simulink model "Ackermann"  (Simulink 8.7)
settings: Solver=ode45  StartTime=0.0  StopTime=10.0  RelTol=1e-3
settings Model: Creator=scaife  LastModifiedBy=bourbouh  ExtModeAutoUpdateStatusClock=off
settings DataIOCC: SignalLoggingSaveFormat=ModelDataLogs  SignalLoggingName=sigsOut
settings DebuggingCC: SaveWithParameterizedLinksMsg=none  SignalResolutionControl=TryResolveAllWithWarning  MultiTaskDSMMsg=warning  MultiTaskCondExecSysMsg=none  StrictBusMsg=None
settings HardwareCC: TargetUnknown=on
settings SFSimCC: SimParseCustomCode=off
settings GRTTargetCC: GeneratePreprocessorConditionals=Use local settings  CombineOutputUpdateFcns=off  GRTInterface=on

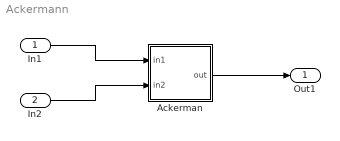
== system Ackermann ==
  In1 : Inport
  In2 : Inport  Port=2
  Ackerman : Stateflow chart  TreatAsAtomicUnit=on
  Out1 : Outport
  wires:
  Ackerman/1(out) -> Out1/1
  In1/1 -> Ackerman/1(in1)
  In2/1 -> Ackerman/2(in2)

== stateflow chart Ackerman ==
  state A/
    entry:
    x[1]=in1;
    y[1]=in2;
    mode[1]=1;
    n=1;
  state B/
    entry:
    out=res[n+1];
  state C/
    entry:
    out=-1;
  (default) -> A
  (junction 15) -> (junction 14) [order 2] : [y[n]==0]
      | {x[n+1]=x[n]-1;
      |  y[n+1]=1;
      |  mode[n+1]=1;
      |  n++;}
  A -> (junction 14)
  (junction 14) -> (junction 15) [order 1] : [x[n]>0]
  (junction 15) -> C [order 3]
  (junction 17) -> (junction 14) [order 3] : [n > 0 & mode[n]==1]
      | {x[n+1]=x[n]-1;
      |  y[n+1]=res[n+1];
      |  mode[n+1]=1;
      |  n++;}
  (junction 15) -> (junction 14) [order 1] : [y[n]>0]
      | {x[n+1]=x[n];
      |  y[n+1]=y[n]-1;
      |  mode[n+1]=2;
      |  n++;}
  (junction 14) -> C [order 3]
  (junction 14) -> (junction 16) [order 2] : [x[n]==0]
      | {res[n]=y[n]+1;
      |  n--;}
  (junction 16) -> (junction 17) [order 1] : [mode[n]>0]
      | {mode[n]--;}
  (junction 16) -> (junction 17) [order 2]
  (junction 17) -> C [order 4]
  (junction 18) -> (junction 17) [order 1] : [mode[n]>0]
      | {mode[n]--;}
  (junction 17) -> B [order 1] : [n==0]
  (junction 17) -> (junction 18) [order 2] : [n>0 & mode[n]==0]
      | {res[n]=res[n+1];
      |  n--;}
  (junction 18) -> (junction 17) [order 2]
  data: x local uint32 size=10; y local uint32 size=10; n local uint32; mode local uint32 size=10; res local uint32 size=10; in1 input uint32; in2 input uint32; out output uint32
